simulink model "BMS_M0_pack_withoutcharging"  (R2026a)
settings: Solver=VariableStepAuto  AbsTol=1e-3  EnableMultiTasking=on
undefined symbols (not defined in the file or in its folder): bat, mcu
libraries: fl_lib x23, nesl_utility x19, batteryecm_lib x6, ee_lib x4, simulink x1
settings SimscapeCC: SimscapeNominalValues="[{\"value\":\"1\",\"unit\":\"A\"},{\"value\":\"1\",\"unit\":\"bar\"},{\"value\":\"1\",\"unit\":\"cm^2\"},{\"value\":\"1\",\"unit\":\"cm^3/s\"},{\"value\":\"1\",\"unit\":\"kJ/kg\"},{\"value\":\"1\",\"unit\":\"kW\"},{\"value\":\"1\",\"unit\":\"l\"},{\"value\":\"1\",\"unit\":\"N\"},{\"value\":\"1\",\"unit\":\"N*m\"},{\"value\":\"1\",\"unit\":\"V\"}]"

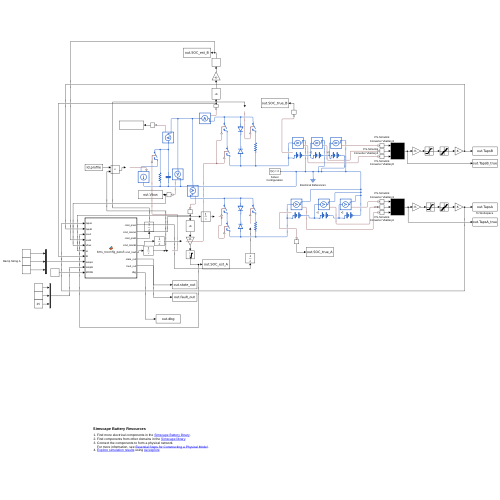
[thumbnail: Simulink's stored preview of the top-level diagram]
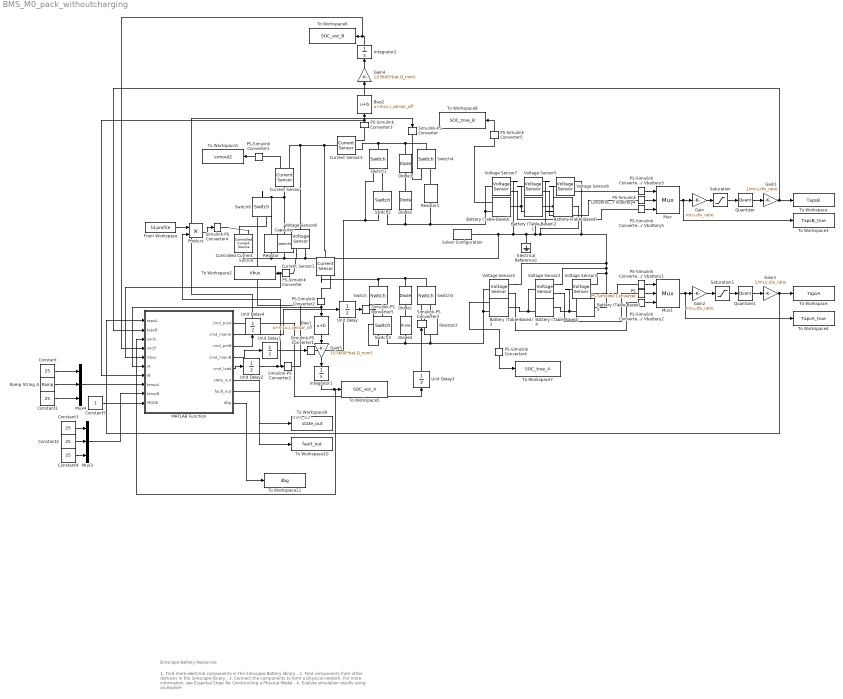
== system BMS_M0_pack_withoutcharging ==
  note: 1. Find more electrical components in the Simscape Battery library .
      | 2. Find components from other domains in the Simscape library .
      | 3. Connect the components to form a physical network.
      | For more information, see Essential Steps for Constructing a Physical Model .
      | 4. Explore simulation results using sscexplore
  note: Simscape Battery Resources
  note: state_out
  Battery (Table-Based){,1..5} (6 alike) : batteryecm_lib/Battery (Table-Based)  SOC_vec=bat.SOC_bp  T_dependence=simscape.enum.tablebattery.temperature_dependence.no  prm_dir=simscape.enum.tablebattery.prm_dir.noCurrentDirectionality  T_vec=[278, 293, 313] K  V0_mat=[3.49, 3.5, 3.51; 3.55, 3.57, 3.56; 3.62, 3.63, 3.64; 3.71, 3.71, 3.72; 3.91, 3.93, 3.94; 4.07, 4.08, 4.08; 4.19, 4.19, 4.19] V  V0_vec=bat.OCV_tbl V  V_range=[0, inf] V  R0_mat=[.0117, .0085, .009; .011, .0085, .009; .0114, .0087, .0092; .0107, .0082, .0088; .0107, .0083, .0091; .0113, .0085, .0089; .0116, .0085, .0089] Ohm  R0_vec=bat.R0 * ones(size(bat.SOC_bp)) Ohm  R0_dis_mat=[.0117, .0085, .009; .011, .0085, .009; .0114, .0087, .0092; .0107, .0082, .0088; .0107, .0083, .0091; .0113, .0085, .0089; .0116, .0085, .0089] Ohm  R0_dis_vec=[.0085, .0085, .0087, .0082, .0083, .0085, .0085] Ohm  R0_ch_mat=[.0117, .0085, .009; .011, .0085, .009; .0114, .0087, .0092; .0107, .0082, .0088; .0107, .0083, .0091; .0113, .0085, .0089; .0116, .0085, .0089] Ohm  R0_ch_vec=[.0085, .0085, .0087, .0082, .0083, .0085, .0085] Ohm  AH=bat.Q_nom A*hr  prm_leak=simscape.enum.tablebattery.prm_leak.disabled  Rleak_vec=[8000, 7000, 6000] Ohm  Rleak=7e3 Ohm  extrapolation_option=simscape.enum.extrapolation.nearest  SOC_port=simscape.enum.tablebattery.enable.yes  prm_dyn=simscape.enum.tablebattery.prm_dyn.off  R1_mat=[.0109, .0029, .0013; .0069, .0024, .0012; .0047, .0026, .0013; .0034, .0016, .001; .0033, .0023, .0014; .0033, .0018, .0011; .0028, .0017, .0011] Ohm  R1_vec=[.0029, .0024, .0026, .0016, .0023, .0018, .0017] Ohm  tau1_mat=[20, 36, 39; 31, 45, 39; 109, 105, 61; 36, 29, 26; 59, 77, 67; 40, 33, 29; 25, 39, 33] s  tau1_vec=[36, 45, 105, 29, 77, 33, 39] s  R2_mat=[.0109, .0029, .0013; .0069, .0024, .0012; .0047, .0026, .0013; .0034, .0016, .001; .0033, .0023, .0014; .0033, .0018, .0011; .0028, .0017, .0011] Ohm  R2_vec=[.0029, .0024, .0026, .0016, .0023, .0018, .0017] Ohm  tau2_mat=[20, 36, 39; 31, 45, 39; 109, 105, 61; 36, 29, 26; 59, 77, 67; 40, 33, 29; 25, 39, 33] s  tau2_vec=[36, 45, 105, 29, 77, 33, 39] s  R3_mat=[.0109, .0029, .0013; .0069, .0024, .0012; .0047, .0026, .0013; .0034, .0016, .001; .0033, .0023, .0014; .0033, .0018, .0011; .0028, .0017, .0011] Ohm  R3_vec=[.0029, .0024, .0026, .0016, .0023, .0018, .0017] Ohm  tau3_mat=[20, 36, 39; 31, 45, 39; 109, 105, 61; 36, 29, 26; 59, 77, 67; 40, 33, 29; 25, 39, 33] s  tau3_vec=[36, 45, 105, 29, 77, 33, 39] s  R4_mat=[.0109, .0029, .0013; .0069, .0024, .0012; .0047, .0026, .0013; .0034, .0016, .001; .0033, .0023, .0014; .0033, .0018, .0011; .0028, .0017, .0011] Ohm  R4_vec=[.0029, .0024, .0026, .0016, .0023, .0018, .0017] Ohm  tau4_mat=[20, 36, 39; 31, 45, 39; 109, 105, 61; 36, 29, 26; 59, 77, 67; 40, 33, 29; 25, 39, 33] s  tau4_vec=[36, 45, 105, 29, 77, 33, 39] s  R5_mat=[.0109, .0029, .0013; .0069, .0024, .0012; .0047, .0026, .0013; .0034, .0016, .001; .0033, .0023, .0014; .0033, .0018, .0011; .0028, .0017, .0011] Ohm  R5_vec=[.0029, .0024, .0026, .0016, .0023, .0018, .0017] Ohm  tau5_mat=[20, 36, 39; 31, 45, 39; 109, 105, 61; 36, 29, 26; 59, 77, 67; 40, 33, 29; 25, 39, 33] s  tau5_vec=[36, 45, 105, 29, 77, 33, 39] s  prm_fade=simscape.enum.tablebattery.prm_fade.disabled  N0=100  dV0=0  dR0=0  dAH=0  dRleak=0  dR1=0  dR2=0  dR3=0  dR4=0  dR5=0  N0vec=[0, 100, 200, 300]  Tfadevec=[298.15, 323.15] K  dV0vec=[0, 0, 0, 0]  dR0vec=[0, 0, 0, 0]  dAHvec=[0, 0, 0, 0]  dRleakvec=[0, 0, 0, 0]  dR1vec=[0, 0, 0, 0]  dR2vec=[0, 0, 0, 0]  dR3vec=[0, 0, 0, 0]  dR4vec=[0, 0, 0, 0]  dR5vec=[0, 0, 0, 0]  dV0mat=[0, 0; 0, 0; 0, 0; 0, 0]  dR0mat=[0, 0; 0, 0; 0, 0; 0, 0]  dAHmat=[0, 0; 0, 0; 0, 0; 0, 0]  dRleakmat=[0, 0; 0, 0; 0, 0; 0, 0]  dR1mat=[0, 0; 0, 0; 0, 0; 0, 0]  dR2mat=[0, 0; 0, 0; 0, 0; 0, 0]  dR3mat=[0, 0; 0, 0; 0, 0; 0, 0]  dR4mat=[0, 0; 0, 0; 0, 0; 0, 0]  dR5mat=[0, 0; 0, 0; 0, 0; 0, 0]  prm_age_modeling=simscape.enum.tablebattery.prm_age_modeling.equation  storage_dt_age_vec=[0] d  storage_T_age_vec=[273] K  prm_age_OCV=simscape.enum.tablebattery.prm_age_OCV.OCV  OCV_age=0.9  SOC_age=0.6  prm_age_resistance=simscape.enum.tablebattery.prm_age.disabled  OCV_scaling_age_resistance=2.2134e6  OCV_offset_age_resistance=1.632e6  temp_exp_age_resistance=0.515833569 V  t_exp_age_resistance=0.75  T_age_vec_resistance=[273.15, 298.15, 323.15] K  dt_age_vec_resistance=[0, 90, 180, 270] d  dR0_age_vec=[0, 0, 0]  t_meas_dR0_age=100 d  dR0_age_mat=[0, 0, 0; 0, 0, 0; 0, 0, 0; 0, 0, 0]  prm_age_capacity=simscape.enum.tablebattery.prm_age.disabled  OCV_scaling_age_capacity=1.5097e07  OCV_offset_age_capacity=8.3625e06  temp_exp_age_capacity=0.6011 V  t_exp_age_capacity=0.75  T_age_vec_capacity=[273.15, 298.15, 323.15] K  dt_age_vec_capacity=[0, 90, 180, 270] d  dAH_age_vec=[0, 0, 0]  t_meas_dAH_age=100 d  dAH_age_mat=[0, 0, 0; 0, 0, 0; 0, 0, 0; 0, 0, 0]  thermal_port=simscape.enum.thermaleffects.omit  temperature=298.15 K  thermal_mass=100 J/K  i_specify=off  i_priority=None  i=0 A  i_nominal_specify=off  i_nominal_value=1  i_nominal_unit=A  v_specify=off  v_priority=None  v=0 V  v_nominal_specify=off  v_nominal_value=1  v_nominal_unit=V  stateOfCharge_specify=on  stateOfCharge_priority=High  stateOfCharge=0.50  stateOfCharge_nominal_specify=off  stateOfCharge_nominal_value=1  stateOfCharge_nominal_unit=1  num_cycles_specify=off  num_cycles_priority=High  num_cycles=0  num_cycles_nominal_specify=off  num_cycles_nominal_value=1  num_cycles_nominal_unit=1  cell_temperature_specify=off  cell_temperature_priority=High  cell_temperature=298.15 K  cell_temperature_nominal_specify=off  cell_temperature_nominal_value=1  cell_temperature_nominal_unit=K
      settings: LibrarySourceBlock=|
      | batt_lib/Cells/Battery
      | (Table-Based)
  Bias1 : Bias  Bias=mcu.i_sensor_off  SaturateOnIntegerOverflow=off
  Bias2 : Bias  Bias=mcu.i_sensor_off  SaturateOnIntegerOverflow=off
  Capacitor : fl_lib/Electrical/Electrical Elements/Capacitor  c=1000 uF  r=1e-6 Ohm  g=0 1/Ohm  i_specify=off  i_priority=None  i=0 A  i_nominal_specify=off  i_nominal_value=1  i_nominal_unit=A  v_specify=off  v_priority=None  v=0 V  v_nominal_specify=off  v_nominal_value=1  v_nominal_unit=V  vc_specify=off  vc_priority=High  vc=0 V  vc_nominal_specify=off  vc_nominal_value=1  vc_nominal_unit=V
  Constant{,1..4} (5 alike) : Constant  Value=25
  Constant5 : Constant
  Controlled Current Source : fl_lib/Electrical/Electrical Sources/Controlled Current Source
  Current Sensor : fl_lib/Electrical/Electrical Sensors/Current Sensor
  Current Sensor1 : fl_lib/Electrical/Electrical Sensors/Current Sensor
  Current Sensor3 : fl_lib/Electrical/Electrical Sensors/Current Sensor
  Diode{1..4} (4 alike) : ee_lib/Semiconductors & Converters/Diode  ModelType=ee.enum.diode.modelType.pwl  TableType=ee.enum.diode.tableType.IfMat  IfMat=[.07, .12, .19, 1.75, 4.24, 7.32, 11.2; .16, .3, .72, 2.14, 5.02, 8.35, 13.12] A  VfMat=[.9, 1.15, 1.25, 1.5, 1.75, 2.17, 2.6, 2.85; .58, .68, .75, 1.1, 1.38, 1.77, 2.27, 2.7] V  TjVec=[25, 125] degC  VfVec=[.5, .7, .9, 1.3, 1.7, 2.1, 2.5] V  IfVec=[.1, .2, .5, 1, 2, 4, 7, 10] A  IrMat=[1e-06, 2e-06, 5e-06, 1e-05, 2.5e-05, 5e-05, .0001; 2e-06, 5e-06, 1e-05, 4e-05, 8e-05, .0002, .0005] A  VrMat=[10, 100, 200, 250, 300, 325, 350; 10, 70, 160, 220, 270, 300, 320] V  VrVec=[10, 20, 40, 50, 70, 80, 100] V  IrVec=[1e-06, 2e-06, 5e-06, 1e-05, 2e-05, 5e-05, .0001] A  Vf=0.8 V  Ron=0.01 Ohm  Goff=1e-8 S  prmExp=ee.enum.diode.expParam.useTwo  I12=[.0137, .545] A  V12=[.6, .7] V  RS=0 Ohm  Tmeas=298.15 K  IS=1e-12 A  ec=1  I1=0.0137 A  V1=0.6 V  N_series=1  N_parallel=1  ZenerEnable=false  Rz=0.3 Ohm  BV=30 V  C_param=ee.enum.diode.capParam.fixed  CJ=0 pF  CJ0=5 pF  Vvec=[.1, 10, 100] V  Cvec=[3.5, 1, .4] pF  VJ=1 V  Mgrad=0.5  FC=0.5  Q_param=ee.enum.diode.recoveryParam.off  iRM=-7.15 A  iF=4 A  didt=-750 A/us  trr_factor=3  trr=115 ns  Qrr=150 nA*s  Vr=-600 V  Ls=150 nH  Erec=0.03 J  TT=50 ns  tau=100 ns  T_param=ee.enum.diode.temperatureParam.off  Tdevice=298.15 K  I1_T2=0.245 A  V1_T2=0.5 V  IS_T2=1.25e-7 A  Tmeas2=125 degC  XTI_param=ee.enum.diode.xtiParam.pn  XTI=3  EG_param=ee.enum.diode.egapParam.material_si  EG=1.11 eV  dBVdT=0 V/K  enable_fault_input=simscape.enum.onoff.off  i_specify=off  i_priority=None  i=0 A  i_nominal_specify=off  i_nominal_value=1  i_nominal_unit=A  v_specify=off  v_priority=None  v=0 V  v_nominal_specify=off  v_nominal_value=1  v_nominal_unit=V  v_capacitor_specify=off  v_capacitor_priority=None  v_capacitor=0 V  v_capacitor_nominal_specify=off  v_capacitor_nominal_value=1  v_capacitor_nominal_unit=V  Qj_specify=off  Qj_priority=High  Qj=0 C  Qj_nominal_specify=off  Qj_nominal_value=1  Qj_nominal_unit=C  i_diode_specify=off  i_diode_priority=None  i_diode=0 A  i_diode_nominal_specify=off  i_diode_nominal_value=1  i_diode_nominal_unit=A  v_diode_specify=off  v_diode_priority=None  v_diode=0 V  v_diode_nominal_specify=off  v_diode_nominal_value=1  v_diode_nominal_unit=V  i_capacitor_specify=off  i_capacitor_priority=None  i_capacitor=0 A  i_capacitor_nominal_specify=off  i_capacitor_nominal_value=1  i_capacitor_nominal_unit=A  fidelity_level=ee.enum.diode.fidelity.includeChargeDyn  rec_loss_model=ee.enum.diode.reverseRecoveryModelTabulateUpTo3D.fixed  ErecVal=0 J  scaleWithIandV=true  ErecMat=zeros(2, 3) J  ErecMat3D=zeros(2, 3, 2) J  TjrecVec=[298.15, 398.15] K  IfrecVec=[.1, 1, 10] A  IrecVal=10 A  VrecVal=10 V  VrecVec=[0, 100] V  tFilter=1 / 1000 / 100 s  thermal_network_parameterization=ee.enum.thermalNetworkTopology.junctionCase  Rth=[0, 10] K/W  Rth_Cauer=[1, 3, 10] K/W  Rth_Foster=[.08, .14, .22, .16] K/W  thermal_mass_parameterization=ee.enum.thermalNetwork.timeconstant  thermal_mass=[0, 1] J/K  thermal_mass_Cauer=[.1, .3, 1] J/K  thermal_mass_Foster=[.001, .005, .05, .5] J/K  thermal_time_constant=[0, 10] s  thermal_time_constant_Cauer=[1, 3, 10] s  thermal_time_constant_Foster=[7e-05, .0007, .01, .08] s  thermal_mass_initial_temperatures=[25, 25] degC  thermal_mass_initial_temperatures_Cauer=[25, 25, 25] degC  junction_thermal_mass=0.01 J/K  Tvec_initial_Foster=[25, 25, 25, 25] degC  no_thermal_network=0  junction_temperature_specify=off  junction_temperature_priority=None  junction_temperature=25 degC  junction_temperature_nominal_specify=off  junction_temperature_nominal_value=1  junction_temperature_nominal_unit=degC
  Electrical Reference1 : fl_lib/Electrical/Electrical Elements/Electrical Reference
  From Workspace : FromWorkspace  VariableName=ld.profile
  Gain : Gain  Gain=mcu.div_ratio
  Gain1 : Gain  Gain=1/mcu.div_ratio
  Gain2 : Gain  Gain=mcu.div_ratio
  Gain3 : Gain  Gain=1/mcu.div_ratio
  Gain4 : Gain  Gain=1/(3600*bat.Q_nom)
  Gain5 : Gain  Gain=1/(3600*bat.Q_nom)
  Integrator1 : Integrator  InitialCondition=0.55  LimitOutput=on  UpperSaturationLimit=1  LowerSaturationLimit=0
  Integrator2 : Integrator  InitialCondition=0.55  LimitOutput=on  UpperSaturationLimit=1  LowerSaturationLimit=0
  MATLAB Function : MATLAB Function  TreatAsAtomicUnit=on  SystemSampleTime=0.1
  Mux{,1,3..4} (4 alike) : Mux  Inputs=3
  PS : nesl_utility/PS-Simulink Converter  PhysicalDomain=network_engine_domain  SubClassName=ps_output  LeftPortType=input  RightPortType=output  PseudoPeriodic=off  Frequencies=[]  VectorFormat=inherit  Unit=inherit  AffineConversion=off
  PS-Simulink Converter{,1..5} (6 alike) : nesl_utility/PS-Simulink Converter  PhysicalDomain=network_engine_domain  SubClassName=ps_output  LeftPortType=input  RightPortType=output  PseudoPeriodic=off  Frequencies=[]  VectorFormat=inherit  Unit=inherit  AffineConversion=off
  PS-Simulink Converter Vbattery{1..5} (5 alike) : nesl_utility/PS-Simulink Converter  PhysicalDomain=network_engine_domain  SubClassName=ps_output  LeftPortType=input  RightPortType=output  PseudoPeriodic=off  Frequencies=[]  VectorFormat=inherit  Unit=inherit  AffineConversion=off
  Product : Product
  Quantizer : Quantizer  QuantizationInterval=mcu.lsb_adc
  Quantizer1 : Quantizer  QuantizationInterval=mcu.lsb_adc
  Ramp String A : simulink/Sources/Ramp  slope=5/60  start=1e9  InitialOutput=25
  Resistor : fl_lib/Electrical/Electrical Elements/Resistor  R=1 MOhm  i_specify=off  i_priority=None  i=0 A  i_nominal_specify=off  i_nominal_value=1  i_nominal_unit=A  v_specify=off  v_priority=None  v=0 V  v_nominal_specify=off  v_nominal_value=1  v_nominal_unit=V
  Resistor1 : fl_lib/Electrical/Electrical Elements/Resistor  R=10 Ohm  i_specify=off  i_priority=None  i=0 A  i_nominal_specify=off  i_nominal_value=1  i_nominal_unit=A  v_specify=off  v_priority=None  v=0 V  v_nominal_specify=off  v_nominal_value=1  v_nominal_unit=V
  Resistor2 : fl_lib/Electrical/Electrical Elements/Resistor  R=10 Ohm  i_specify=off  i_priority=None  i=0 A  i_nominal_specify=off  i_nominal_value=1  i_nominal_unit=A  v_specify=off  v_priority=None  v=0 V  v_nominal_specify=off  v_nominal_value=1  v_nominal_unit=V
  Saturation : Saturate  UpperLimit=3.3  LowerLimit=0
  Saturation1 : Saturate  UpperLimit=3.3  LowerLimit=0
  Simulink-PS Converter{,1..5} (6 alike) : nesl_utility/Simulink-PS Converter  PhysicalDomain=network_engine_domain  SubClassName=ps_input  LeftPortType=input  RightPortType=output  PseudoPeriodic=off  Frequencies=[]  NoiseDistribution=none  NoiseParameters=[]  Unit=1  AffineConversion=off  FilteringAndDerivatives=provide  SimscapeFilterOrder=1  InputFilterTimeConstant=0.001  UdotUserProvided=0
  Solver Configuration : nesl_utility/Solver Configuration  PhysicalDomain=network_engine_domain  SubClassName=solver  LeftPortType=input  RightPortType=generic  Tones=[]  Harmonics=[]  SimulateNoise=off  Profile=off  UseLocalSampling=off  EnableSwitchedLinearOptims=on  FrequencyDomain=off  UseCCode=off  RelTol=0.001  AbsTol=1e-06  MinStep=1e-09  ToWorkspace=off  RevertToSquareIcSolve=off  NumHomotopyIterations=100  PhasorMode=off  PhasorModeNumHarmonics=1  ConsistencySolver=NEWTON_XTOL_AFTER_FTOL  CanonicalOrdering=UNORDERED  OptimizeIntermediates=UNOPTIMIZED  IndexReductionMethod=DerivativeReplacement  DoDC=off  ResidualTolerance=1e-09  ConsistencyTolSource=GLOBAL  ConsistencyAbsTol=0.001  ConsistencyRelTol=0.001  ConsistencyTolFactor=0.001  UseLocalSolver=off  LocalSolverChoice=NE_BACKWARD_EULER_ADVANCER  ResolveIndetEquations=on  FunctionEvalNumThread=1  LocalSolverSampleTime=0.001  DoFixedCost=off  MaxNonlinIter=3  MaxModeIter=2  ComputeImpulses=off  ImpulseIterations=2  LinearAlgebra=auto  LinearAlgebraNumThread=0  EquationFormulation=NE_TIME_EF  DelaysMemoryBudget=1024  AutomaticFiltering=on  FilteringTimeConstant=0.001  PartitionStorageMethod=AS_NEEDED  PartitionMemoryBudget=1024  PartitionMethod=ROBUST  MultibodyUseLocalSolver=off  MultibodyLocalSolverChoice=ODE1  MultibodyLocalSolverSampleTime=0.001
  Switch{,1..3,6} (5 alike) : fl_lib/Electrical/Electrical Elements/Switch  R_closed=fet.Rds_on Ohm  G_open=1e-8 1/Ohm  Threshold=0.5  i_specify=off  i_priority=None  i=0 A  i_nominal_specify=off  i_nominal_value=1  i_nominal_unit=A  v_specify=off  v_priority=None  v=0 V  v_nominal_specify=off  v_nominal_value=1  v_nominal_unit=V
  Switch4 : fl_lib/Electrical/Electrical Elements/Switch  R_closed=0.01 Ohm  G_open=1e-8 1/Ohm  Threshold=0.5  i_specify=off  i_priority=None  i=0 A  i_nominal_specify=off  i_nominal_value=1  i_nominal_unit=A  v_specify=off  v_priority=None  v=0 V  v_nominal_specify=off  v_nominal_value=1  v_nominal_unit=V
  Switch5 : fl_lib/Electrical/Electrical Elements/Switch  R_closed=0.01 Ohm  G_open=1e-8 1/Ohm  Threshold=0.5  i_specify=off  i_priority=None  i=0 A  i_nominal_specify=off  i_nominal_value=1  i_nominal_unit=A  v_specify=off  v_priority=None  v=0 V  v_nominal_specify=off  v_nominal_value=1  v_nominal_unit=V
  To Workspace : ToWorkspace  VariableName=TapsB  SaveFormat=Timeseries  SampleTime=-1
  "To Workspace " : ToWorkspace  VariableName=TapsA  SaveFormat=Timeseries  SampleTime=-1
  To Workspace1 : ToWorkspace  VariableName=simout2  SaveFormat=Timeseries  SampleTime=-1
  To Workspace10 : ToWorkspace  VariableName=fault_out  SaveFormat=Timeseries  SampleTime=-1
  To Workspace11 : ToWorkspace  VariableName=dbg  SaveFormat=Timeseries  SampleTime=-1
  To Workspace2 : ToWorkspace  VariableName=Vbus  SaveFormat=Timeseries  SampleTime=-1
  To Workspace3 : ToWorkspace  VariableName=TapsB_true  SaveFormat=Timeseries  SampleTime=-1
  To Workspace4 : ToWorkspace  VariableName=TapsA_true  SaveFormat=Timeseries  SampleTime=-1
  To Workspace5 : ToWorkspace  VariableName=SOC_est_A  SaveFormat=Timeseries  SampleTime=-1
  To Workspace6 : ToWorkspace  VariableName=SOC_est_B  SaveFormat=Timeseries  SampleTime=-1
  To Workspace7 : ToWorkspace  VariableName=SOC_true_A  SaveFormat=Timeseries  SampleTime=-1
  To Workspace8 : ToWorkspace  VariableName=SOC_true_B  SaveFormat=Timeseries  SampleTime=-1
  To Workspace9 : ToWorkspace  VariableName=state_out  SaveFormat=Timeseries  SampleTime=-1
  Unit Delay{,1..4} (5 alike) : UnitDelay  SampleTime=0.1
  Voltage Sensor{2..8} (7 alike) : fl_lib/Electrical/Electrical Sensors/Voltage Sensor
  wires:
  Saturation1/1 -> Quantizer1/1
  Unit Delay2/1 -> Product/2, Simulink-PS Converter2/1
  PS-Simulink Converter3/1 -> MATLAB Function/7(iB), Bias2/1
  Mux4/1 -> MATLAB Function/8(tempA)
  MATLAB Function/8(dbg) -> To Workspace11/1
  Constant1/1 -> Mux4/3
  Constant5/1 -> MATLAB Function/10(MODE)
  Unit Delay/1 -> Simulink-PS Converter5/1
  PS-Simulink Converter Vbattery3/1 -> Mux/1
  MATLAB Function/4(cmd_mainB) -> Unit Delay1/1
  PS-Simulink Converter Vbattery1/1 -> Mux1/1
  Ramp String A/1 -> Mux4/2
  Constant/1 -> Mux4/1
  Constant4/1 -> Mux3/3
  PS-Simulink Converter/1 -> To Workspace2/1, MATLAB Function/5(Vbus)
  PS-Simulink Converter2/1 -> MATLAB Function/6(iA), Bias1/1
  Product/1 -> Simulink-PS Converter4/1
  Quantizer1/1 -> Gain3/1
  MATLAB Function/3(cmd_preB) -> Unit Delay4/1
  Gain/1 -> Saturation/1
  PS-Simulink Converter5/1 -> To Workspace8/1
  Quantizer/1 -> Gain1/1
  Constant3/1 -> Mux3/1
  PS-Simulink Converter Vbattery5/1 -> Mux/3
  Integrator2/1 -> MATLAB Function/4(socB), To Workspace6/1
  Saturation/1 -> Quantizer/1
  Bias2/1 -> Gain4/1
  Integrator1/1 -> To Workspace5/1, MATLAB Function/3(socA)
  Unit Delay3/1 -> Simulink-PS Converter3/1
  Mux3/1 -> MATLAB Function/9(tempB)
  PS-Simulink Converter1/1 -> To Workspace1/1
  MATLAB Function/5(cmd_load) -> Unit Delay2/1
  MATLAB Function/6(state_out) -> To Workspace9/1
  MATLAB Function/2(cmd_mainA) -> Unit Delay/1
  Gain5/1 -> Integrator1/1
  PS-Simulink Converter Vbattery4/1 -> Mux/2
  From Workspace/1 -> Product/1
  Gain1/1 -> To Workspace/1, MATLAB Function/2(tapsB)
  Gain4/1 -> Integrator2/1
  Gain3/1 -> "To Workspace "/1, MATLAB Function/1(tapsA)
  Constant2/1 -> Mux3/2
  PS-Simulink Converter Vbattery2/1 -> Mux1/3
  Unit Delay1/1 -> Simulink-PS Converter1/1
  PS-Simulink Converter4/1 -> To Workspace7/1
  PS/1 -> Mux1/2
  Mux/1 -> To Workspace3/1, Gain/1
  Gain2/1 -> Saturation1/1
  MATLAB Function/7(fault_out) -> To Workspace10/1
  MATLAB Function/1(cmd_preA) -> Unit Delay3/1
  Mux1/1 -> To Workspace4/1, Gain2/1
  Unit Delay4/1 -> Simulink-PS Converter/1
  Bias1/1 -> Gain5/1
  connections:
  Voltage Sensor6/RConn2 -- Battery (Table-Based)5/RConn1 -- Voltage Sensor3/RConn2 -- Voltage Sensor2/RConn2 -- Voltage Sensor4/RConn2 -- Solver Configuration/RConn1 -- Controlled Current Source/LConn1 -- Resistor/RConn1 -- Capacitor/RConn1 -- Voltage Sensor8/RConn2 -- Voltage Sensor7/RConn2 -- Electrical Reference1/LConn1 -- Voltage Sensor5/RConn2 -- Battery (Table-Based)2/RConn1
  Diode1/LConn1 -- Switch/LConn1 -- Current Sensor1/RConn2 -- Switch5/LConn1
  Current Sensor3/RConn2 -- Switch1/LConn1 -- Switch4/LConn1 -- Diode3/LConn1
  Switch/RConn1 -- Simulink-PS Converter5/RConn1 -- Switch3/RConn1
  Battery (Table-Based)2/LConn1 -- Battery (Table-Based)1/RConn1 -- Voltage Sensor6/LConn1
  Battery (Table-Based)5/LConn1 -- Battery (Table-Based)4/RConn1 -- Voltage Sensor3/LConn1
  Diode2/LConn1 -- Switch2/RConn2 -- Resistor1/RConn1 -- Voltage Sensor7/LConn1 -- Battery (Table-Based)/LConn1
  Switch2/RConn1 -- Simulink-PS Converter1/RConn1 -- Switch1/RConn1
  Current Sensor/RConn2 -- Current Sensor3/LConn1 -- Current Sensor1/LConn1 -- Voltage Sensor8/LConn1
  Voltage Sensor4/LConn1 -- Resistor2/RConn1 -- Diode4/LConn1 -- Switch3/RConn2 -- Battery (Table-Based)3/LConn1
  Battery (Table-Based)4/LConn1 -- Battery (Table-Based)3/RConn1 -- Voltage Sensor2/LConn1
  Switch6/LConn1 -- Capacitor/LConn1 -- Current Sensor/LConn1 -- Resistor/LConn1
  Voltage Sensor5/LConn1 -- Battery (Table-Based)/RConn1 -- Battery (Table-Based)1/LConn1
  Voltage Sensor6/RConn1 -- PS-Simulink Converter Vbattery3/LConn1
  Simulink-PS Converter3/RConn1 -- Switch5/RConn1
  Switch1/RConn2 -- Switch2/LConn1
  Current Sensor3/RConn1 -- PS-Simulink Converter3/LConn1
  Voltage Sensor4/RConn1 -- PS-Simulink Converter Vbattery2/LConn1
  Current Sensor/RConn1 -- PS-Simulink Converter1/LConn1
  Resistor1/LConn1 -- Switch4/RConn2
  Voltage Sensor8/RConn1 -- PS-Simulink Converter/LConn1
  Switch6/RConn2 -- Controlled Current Source/RConn2
  Switch/RConn2 -- Switch3/LConn1
  Simulink-PS Converter2/RConn1 -- Switch6/RConn1
  PS-Simulink Converter4/LConn1 -- Battery (Table-Based)3/LConn2
  Simulink-PS Converter4/RConn1 -- Controlled Current Source/RConn1
  Voltage Sensor5/RConn1 -- PS-Simulink Converter Vbattery4/LConn1
  Diode4/RConn1 -- Diode1/RConn1
  Resistor2/LConn1 -- Switch5/RConn2
  Voltage Sensor3/RConn1 -- PS-Simulink Converter Vbattery1/LConn1
  Voltage Sensor2/RConn1 -- PS/LConn1
  Current Sensor1/RConn1 -- PS-Simulink Converter2/LConn1
  Voltage Sensor7/RConn1 -- PS-Simulink Converter Vbattery5/LConn1
  Battery (Table-Based)/LConn2 -- PS-Simulink Converter5/LConn1
  Diode2/RConn1 -- Diode3/RConn1
  Switch4/RConn1 -- Simulink-PS Converter/RConn1

== matlab function BMS_M0_pack_withoutcharging/MATLAB Function ==
  data: cmd_preA output; tapsA input; cmd_mainA output; cmd_preB output; tapsB input; socA input; socB input; cmd_mainB output; cmd_load output; state_out output; fault_out output; Vbus input; iA input; iB input; dbg output; tempA input; tempB input; MODE input
function [cmd_preA, cmd_mainA, cmd_preB, cmd_mainB, cmd_load, ...
          state_out, fault_out, dbg] = ...
         bms_reconfig_pass5(tapsA, tapsB, socA, socB, Vbus, iA, iB, ...
                            tempA, tempB, MODE)
%BMS_RECONFIG_PASS5  SOC/SOA-driven string-level reconfiguration controller.
%
%  ====================================================================
%  PROPRIETARY -- this file contains the novel contribution of this
%  project: dynamic string connect/disconnect/precharge for fault
%  isolation and SOC-driven wear levelling in a reconfigurable 3S2P pack.
%  Do not paste this logic into generic BMS code templates.
%  ====================================================================
%
%  MILESTONE 0 -- PASS 5 (final for M0).
%
%  REVISION HISTORY
%    Rev 1  SOA + topology logic.
%    Rev 2  Weld detection gated on precharge (Rev 1 tripped F_WELD_A on
%           startup because precharge current flows while the main pair is
%           deliberately open). SOC rejoin hysteresis actually applied --
%           Rev 1 rejoined at gap <= SPLIT_TH instead of < REJOIN_TH, so
%           the hysteresis band did nothing.
%    Rev 3  Warm-parallel guard reformulated. The 0.1 V rule is retained
%           for cold start, but under load the terminal difference between
%           strings is dominated by IR drop rather than stored-energy
%           mismatch, so it can never be satisfied. Bounded inrush is the
%           physically meaningful criterion. MEASURED Scenario 3: join at
%           dV = 0.149 V, inrush 1.5 A -> I_JOIN_MAX = 6 A gives 4x margin
%           while still blocking the 6.9 A cold-parallel case.
%    Rev 4  Overtemperature added.
%    Rev 5  MODE input added for the Day 5 fixed-vs-reconfigurable
%           comparison. The override MUST sit after the transition switch
%           statement -- an earlier attempt placed it before, where it was
%           silently overwritten by `case S_BOTH` within the same call and
%           the two configurations produced identical results.
%
%  DESIGN RULES (from project brief, enforced in this order):
%    1. SOA checks run BEFORE any efficiency or balancing logic.
%    2. Break-before-make on every topology change.
%    3. Never parallel two strings unless the resulting inrush is bounded
%       (see Rev 3 note -- the original 0.1 V form is kept for cold start).
%    4. Minimum cooldown between topology changes (anti-oscillation).
%    5. Power-up / reset default is ALL SWITCHES OPEN.
%    6. Every switching action is validated by reading back current.
%
%  INPUTS
%    tapsA, tapsB  3x1  quantised tap voltages, referenced to pack negative
%    socA, socB    1x1  COULOMB-COUNTED estimates. Never true SOC.
%    Vbus          1x1  bus voltage (measured)
%    iA, iB        1x1  per-string current (measured, + = discharge)
%    tempA, tempB  3x1  per-cell temperature (deg C).
%                       INJECTED forcing function, not a thermal model --
%                       see M0 Day 1 scope decision. M0 makes NO claim
%                       about temperature reduction; that is bench-measured
%                       in M4.
%    MODE          1x1  0 = fixed-pack baseline, 1 = reconfigurable.
%                       See the MODE block in LAYER 3 for what MODE 0
%                       does and why the comparison is fair.
%
%  OUTPUTS
%    cmd_preA/B    0/1  precharge bypass switch per string
%    cmd_mainA/B   0/1  main back-to-back pair per string
%    cmd_load      0/1  load disconnect switch
%    state_out          state code
%    fault_out          latched fault bitfield
%    dbg          10x1  diagnostics

%% ---- CONSTANTS ------------------------------------------------------
% KEEP IN SYNC WITH BMS_params.m -- a MATLAB Function block cannot read
% the base workspace.
DT              = 0.100;  % s   control loop period
V_UV_TRIP       = 2.50;   % V   [VERIFIED] SPEC pack design guideline, NCA
V_OV_TRIP       = 4.20;   % V   [VERIFIED] SPEC 3.3
I_OC_TRIP       = 12.0;   % A   [ASSUMPTION] per string, below the 15 A
                          %     cell rating with margin
T_OT_TRIP       = 60.0;   % C   [DESIGN] SPEC recommends re-discharge
                          %     release below 60 C. INTRO p.6 shows a 10 A
                          %     discharge reaching 60.9 C -- i.e. exactly
                          %     the single-string fault-mode operating
                          %     point, so this threshold is meaningful
                          %     rather than arbitrary.
T_OT_WARN       = 50.0;   % C   [ASSUMPTION] early-warning margin
DV_PARALLEL_MAX = 0.10;   % V   [ASSUMPTION] cold-start parallel limit
I_JOIN_MAX      = 6.0;    % A   [MEASURED-derived] Scenario 3 joined at
                          %     1.5 A; 6 A is 4x that and still blocks the
                          %     6.9 A unbalanced-warm-join case
R_STRING        = 0.100;  % ohm [CALCULATED] 3*20 mOhm cells + 2*20 mOhm
                          %     back-to-back MOSFET pair
T_COOLDOWN      = 0.50;   % s   [ASSUMPTION] min between topology changes
T_PRECHARGE_MAX = 0.50;   % s   [CALCULATED] 5*tau = 50 ms at R_pre = 10
                          %     ohm, C_bus = 1000 uF; 10x margin
VBUS_PRE_FRAC   = 0.95;   % fraction of string voltage = precharge done
SOC_SPLIT_TH    = 0.15;   % [DESIGN] gap at which we stop paralleling
SOC_REJOIN_TH   = 0.05;   % [DESIGN] hysteresis band for rejoining
DEBOUNCE_N      = 3;      % consecutive samples before a fault latches
VALIDATE_N      = 5;      % samples allowed for a switch to prove it moved
I_CONDUCT_MIN   = 0.20;   % A   above this counts as "current flowing"
STARTUP_N       = 10;     % ignore SOA for first 1 s while Simscape settles

%% ---- STATE CODES ----------------------------------------------------
S_INIT     = 0;   S_PRE_A    = 1;   S_PRE_B    = 2;
S_SINGLE_A = 3;   S_SINGLE_B = 4;   S_BOTH     = 5;
S_SHUTDOWN = 6;

%% ---- FAULT BITS -----------------------------------------------------
F_NONE   = 0;
F_UV_A   = 1;     F_UV_B   = 2;
F_OV_A   = 4;     F_OV_B   = 8;
F_OC_A   = 16;    F_OC_B   = 32;
F_PRE_A  = 64;    F_PRE_B  = 128;
F_WELD_A = 256;   F_WELD_B = 512;
F_OPEN_A = 1024;  F_OPEN_B = 2048;
F_OT_A   = 4096;  F_OT_B   = 8192;    % overtemperature

%% ---- PERSISTENT STATE ----------------------------------------------
persistent state fault
persistent uvA_c uvB_c ovA_c ovB_c ocA_c ocB_c otA_c otB_c
persistent t_state t_cool startup_c
persistent last_mainA last_mainB last_preA last_preB validate_cA validate_cB

if isempty(state)
    % POWER-UP DEFAULT: everything open. Mirrors the 100k base pull-downs
    % on the 2N2222A drivers -- on reset or brownout the hardware holds
    % the MOSFETs off, and the controller agrees.
    state = S_INIT;  fault = F_NONE;
    uvA_c = 0; uvB_c = 0; ovA_c = 0; ovB_c = 0;
    ocA_c = 0; ocB_c = 0; otA_c = 0; otB_c = 0;
    t_state = 0; t_cool = 0; startup_c = 0;
    last_mainA = 0; last_mainB = 0;
    last_preA  = 0; last_preB  = 0;
    validate_cA = 0; validate_cB = 0;
end

startup_c = startup_c + 1;
t_state   = t_state + DT;
if t_cool > 0, t_cool = t_cool - DT; end

%% ---- RECONSTRUCT PER-CELL VOLTAGES ---------------------------------
% The firmware performs this same subtraction: the dividers measure taps
% relative to pack negative, not individual cells. Measured reconstruction
% error 0.39 mV typical, ~7 mV worst case (2 LSB at 3.46 mV/LSB).
vA = [ tapsA(1); tapsA(2)-tapsA(1); tapsA(3)-tapsA(2) ];
vB = [ tapsB(1); tapsB(2)-tapsB(1); tapsB(3)-tapsB(2) ];

vStringA = tapsA(3);
vStringB = tapsB(3);

tMaxA = max(tempA);
tMaxB = max(tempB);

%% ---- STARTUP GRACE --------------------------------------------------
if startup_c < STARTUP_N
    cmd_preA = 0; cmd_mainA = 0;
    cmd_preB = 0; cmd_mainB = 0; cmd_load = 0;
    state_out = S_INIT; fault_out = F_NONE;
    dbg = [vA(1); vA(2); vA(3); vB(1); vB(2); vB(3); 0; 0; tMaxA; tMaxB];
    return
end

%% =====================================================================
%  LAYER 1 -- SOA CHECKS. These run first, always, and override
%  everything below.
%  =====================================================================
if any(vA < V_UV_TRIP),  uvA_c = uvA_c + 1; else, uvA_c = 0; end
if any(vB < V_UV_TRIP),  uvB_c = uvB_c + 1; else, uvB_c = 0; end
if any(vA > V_OV_TRIP),  ovA_c = ovA_c + 1; else, ovA_c = 0; end
if any(vB > V_OV_TRIP),  ovB_c = ovB_c + 1; else, ovB_c = 0; end
if abs(iA) > I_OC_TRIP,  ocA_c = ocA_c + 1; else, ocA_c = 0; end
if abs(iB) > I_OC_TRIP,  ocB_c = ocB_c + 1; else, ocB_c = 0; end
if tMaxA   > T_OT_TRIP,  otA_c = otA_c + 1; else, otA_c = 0; end
if tMaxB   > T_OT_TRIP,  otB_c = otB_c + 1; else, otB_c = 0; end

% Faults LATCH. An unloaded cell recovers voltage and would look healthy
% again; a cell removed from a heat source cools. Re-closing on either
% would oscillate the pack.
if uvA_c >= DEBOUNCE_N, fault = bitor(fault, F_UV_A); end
if uvB_c >= DEBOUNCE_N, fault = bitor(fault, F_UV_B); end
if ovA_c >= DEBOUNCE_N, fault = bitor(fault, F_OV_A); end
if ovB_c >= DEBOUNCE_N, fault = bitor(fault, F_OV_B); end
if ocA_c >= DEBOUNCE_N, fault = bitor(fault, F_OC_A); end
if ocB_c >= DEBOUNCE_N, fault = bitor(fault, F_OC_B); end
if otA_c >= DEBOUNCE_N, fault = bitor(fault, F_OT_A); end
if otB_c >= DEBOUNCE_N, fault = bitor(fault, F_OT_B); end

%% ---- STATE VALIDATION ----------------------------------------------
% A MOSFET welded closed is invisible to voltage sensing -- only current
% reveals it. Gate on the PREVIOUS cycle's precharge command: while a
% precharge switch is closed the main pair is deliberately open yet
% current legitimately flows through R_pre, which is otherwise
% indistinguishable from a weld.
in_precharge = (last_preA == 1) || (last_preB == 1);

if ~in_precharge && last_mainA == 0 && abs(iA) > I_CONDUCT_MIN
    fault = bitor(fault, F_WELD_A);
end
if ~in_precharge && last_mainB == 0 && abs(iB) > I_CONDUCT_MIN
    fault = bitor(fault, F_WELD_B);
end
% Commanded closed but no current.
% Two fixes from M0 review:
%   (a) Split counters -- shared validate_c cross-contaminated A/B.
%   (b) Gate on evidence that current SHOULD be flowing:
%       S_BOTH:     other string is carrying current (proves load is active)
%       S_SINGLE_X: Vbus not tracking string voltage (proves switch isn't conducting)
%       Without this gate, a healthy no-load idle trips the detector.

i_total = abs(iA) + abs(iB);
vbus_tracks_A = (abs(Vbus - vStringA) < 1.0);
vbus_tracks_B = (abs(Vbus - vStringB) < 1.0);

% --- String A open-wire check ---
openA_cond = false;
if state == S_BOTH && last_mainA == 1 && ...
        abs(iA) < I_CONDUCT_MIN && i_total > I_CONDUCT_MIN && t_state > 1.0
    openA_cond = true;   % load is active but A carries nothing
elseif state == S_SINGLE_A && last_mainA == 1 && ...
        abs(iA) < I_CONDUCT_MIN && ~vbus_tracks_A && t_state > 1.0
    openA_cond = true;   % bus isn't tracking string A despite switch closed
end

if openA_cond
    validate_cA = validate_cA + 1;
    if validate_cA >= VALIDATE_N, fault = bitor(fault, F_OPEN_A); end
else
    validate_cA = 0;
end

% --- String B open-wire check ---
openB_cond = false;
if state == S_BOTH && last_mainB == 1 && ...
        abs(iB) < I_CONDUCT_MIN && i_total > I_CONDUCT_MIN && t_state > 1.0
    openB_cond = true;
elseif state == S_SINGLE_B && last_mainB == 1 && ...
        abs(iB) < I_CONDUCT_MIN && ~vbus_tracks_B && t_state > 1.0
    openB_cond = true;
end

if openB_cond
    validate_cB = validate_cB + 1;
    if validate_cB >= VALIDATE_N, fault = bitor(fault, F_OPEN_B); end
else
    validate_cB = 0;
end

faultA = bitand(fault, F_UV_A + F_OV_A + F_OC_A + F_OT_A + ...
                       F_PRE_A + F_WELD_A + F_OPEN_A) ~= 0;
faultB = bitand(fault, F_UV_B + F_OV_B + F_OC_B + F_OT_B + ...
                       F_PRE_B + F_WELD_B + F_OPEN_B) ~= 0;

%% =====================================================================
%  LAYER 2 -- BALANCING PREFERENCE (secondary; never overrides Layer 1)
%
%  A 2S string cannot be paralleled with a 3S string, so per-cell bypass
%  is unavailable. String-level selection is the only lever: run the
%  fuller string alone and let the emptier one rest.
%
%  MEASURED BEHAVIOUR (Scenario 3): from a 15% gap, single-string
%  operation closed the gap to 5% in 224 s, at which point the strings
%  rejoined. After rejoining the gap continued to zero WITHOUT controller
%  action -- paralleled strings self-balance through the bus. The value of
%  the split is therefore SAFE CONNECTION of mismatched strings, not extra
%  extracted energy. Do not claim the latter.
%  =====================================================================
soc_gap = socA - socB;
prefer_A_only = (soc_gap >  SOC_SPLIT_TH);
prefer_B_only = (soc_gap < -SOC_SPLIT_TH);
rejoin_ok     = (abs(soc_gap) < SOC_REJOIN_TH);

%% =====================================================================
%  LAYER 3 -- TRANSITION GUARDS
%  =====================================================================
% Cold start (load off, bus near 0 V): terminal dV is the right check.
% Warm parallel (load on): terminal dV is dominated by IR drop from the
% loaded string, not by stored-energy mismatch, so it can never fall below
% 0.1 V. Bound the resulting inrush instead -- that is the quantity the
% original rule was a proxy for.
dV_terminal = abs(vStringA - vStringB);
inrush_est  = dV_terminal / R_STRING;
dV_ok       = (dV_terminal < DV_PARALLEL_MAX) || (inrush_est < I_JOIN_MAX);

cool_ok   = (t_cool <= 0);
new_state = state;

switch state

    case S_INIT
        if     faultA && faultB, new_state = S_SHUTDOWN;
        elseif ~faultA,          new_state = S_PRE_A;
        elseif ~faultB,          new_state = S_PRE_B;
        else,                    new_state = S_SHUTDOWN;
        end

    case S_PRE_A
        % Bus charges through R_pre with the load disconnected. Only once
        % it has risen does the main pair close -- this is what keeps the
        % handover near 1 A instead of the measured 219 A cold-connect.
        if faultA
            new_state = S_SHUTDOWN;
        elseif Vbus >= VBUS_PRE_FRAC * vStringA
            new_state = S_SINGLE_A;
        elseif t_state > T_PRECHARGE_MAX
            fault = bitor(fault, F_PRE_A);
            new_state = S_SHUTDOWN;
        end

    case S_PRE_B
        if faultB
            new_state = S_SINGLE_A;
        elseif Vbus >= VBUS_PRE_FRAC * vStringB
            new_state = S_BOTH;
        elseif t_state > T_PRECHARGE_MAX
            fault = bitor(fault, F_PRE_B);
            new_state = S_SINGLE_A;
        end

    case S_SINGLE_A
        if     faultA && faultB,      new_state = S_SHUTDOWN;
        elseif faultA,                new_state = S_PRE_B;
        elseif ~faultB && cool_ok && dV_ok && rejoin_ok
                                      new_state = S_PRE_B;
        end

    case S_SINGLE_B
        if     faultA && faultB,      new_state = S_SHUTDOWN;
        elseif faultB,                new_state = S_PRE_A;
        elseif ~faultA && cool_ok && dV_ok && rejoin_ok
                                      new_state = S_PRE_A;
        end

    case S_BOTH
        if     faultA && faultB,         new_state = S_SHUTDOWN;
        elseif faultA,                   new_state = S_SINGLE_B;
        elseif faultB,                   new_state = S_SINGLE_A;
        elseif cool_ok && prefer_A_only, new_state = S_SINGLE_A;
        elseif cool_ok && prefer_B_only, new_state = S_SINGLE_B;
        end

    case S_SHUTDOWN
        % TERMINAL. Auto-recovery from an unknown fault is not defensible.

    otherwise
        new_state = S_SHUTDOWN;
end

%% ---- MODE 0: FIXED-PACK BASELINE ------------------------------------
% A conventional hard-paralleled pack has no string switches, so it cannot
% isolate a faulted string. Once both strings are connected the topology is
% frozen: faults still latch and are logged, but produce no reconfiguration.
% The only exit is total shutdown once the pack can no longer supply.
%
% Everything else -- cell models, switch resistance, body diodes, sensing,
% quantisation, precharge at startup -- is IDENTICAL to MODE 1. The only
% difference is the control policy, which is exactly what we are comparing.
%
% PLACEMENT MATTERS: this must run AFTER the switch statement above, so it
% overrides the new_state that `case S_BOTH` just computed. Placing it
% before the switch has no effect -- the transition logic simply recomputes
% new_state and the override is lost.
if MODE < 0.5 && state == S_BOTH
    if faultA && faultB
        new_state = S_SHUTDOWN;   % pack exhausted; nothing left to do
    else
        new_state = S_BOTH;       % freeze -- no isolation available
    end
end

if new_state ~= state
    state   = new_state;
    t_state = 0;
    t_cool  = T_COOLDOWN;
end

%% ---- OUTPUTS -------------------------------------------------------
% BREAK-BEFORE-MAKE is structural: no state asserts a precharge switch and
% its own main pair simultaneously.
switch state
    case S_INIT
        cmd_preA=0; cmd_mainA=0; cmd_preB=0; cmd_mainB=0; cmd_load=0;
    case S_PRE_A
        cmd_preA=1; cmd_mainA=0; cmd_preB=0; cmd_mainB=0; cmd_load=0;
    case S_SINGLE_A
        cmd_preA=0; cmd_mainA=1; cmd_preB=0; cmd_mainB=0; cmd_load=1;
    case S_PRE_B
        cmd_preA=0; cmd_mainA=1; cmd_preB=1; cmd_mainB=0; cmd_load=1;
    case S_SINGLE_B
        cmd_preA=0; cmd_mainA=0; cmd_preB=0; cmd_mainB=1; cmd_load=1;
    case S_BOTH
        cmd_preA=0; cmd_mainA=1; cmd_preB=0; cmd_mainB=1; cmd_load=1;
    case S_SHUTDOWN
        cmd_preA=0; cmd_mainA=0; cmd_preB=0; cmd_mainB=0; cmd_load=0;
    otherwise
        cmd_preA=0; cmd_mainA=0; cmd_preB=0; cmd_mainB=0; cmd_load=0;
end

last_mainA = cmd_mainA;  last_mainB = cmd_mainB;
last_preA  = cmd_preA;   last_preB  = cmd_preB;

state_out = state;
fault_out = fault;
dbg = [vA(1); vA(2); vA(3); vB(1); vB(2); vB(3); ...
       soc_gap; Vbus; tMaxA; tMaxB];

end

%% =====================================================================
%  FMEA -- PASS 5
%  =====================================================================
%
%  FAILURE                   DETECTION                   SAFE RESPONSE
%  --------------------------------------------------------------------
%  Cell undervoltage         cell < 2.50 V, 3 samples    Isolate string
%  Cell overvoltage          cell > 4.20 V, 3 samples    Isolate string
%  String overcurrent        |i| > 12 A, 3 samples       Isolate string
%  Cell overtemperature      T > 60 C, 3 samples         Isolate string
%
%  Internal cell short       Manifests as UV on that     Isolate string.
%  (the case a hard-          cell, and/or OT            Series topology
%   paralleled pack                                      means no loop
%   cannot address)                                      exists once the
%                                                        string switch is
%                                                        open. Measured
%                                                        leakage with the
%                                                        pair open:
%                                                        0.0004 mA.
%
%  MOSFET welded closed      commanded open but          Latch F_WELD;
%                            |i| > 0.2 A and not         cannot isolate,
%                            during precharge            so SHUTDOWN via
%                                                        load disconnect
%
%  MOSFET failed open        commanded closed but        Latch F_OPEN,
%                            |i| < 0.2 A, 5 samples      treat string as
%                                                        faulted
%
%  Single switch instead     N/A -- design-time.         MEASURED: a single
%  of a back-to-back pair    Body diode conducts.        switch leaked
%                                                        168,571 mA vs
%                                                        0.0004 mA for the
%                                                        pair. This is why
%                                                        the pair is
%                                                        mandatory.
%
%  Precharge resistor open   Vbus below 95% after        Latch F_PRE; do
%                            500 ms                      not close the main
%                                                        pair. Prevents the
%                                                        measured 218.8 A
%                                                        cold-connect.
%
%  Precharge switch welded   R_pre dissipates            NOT DETECTED.
%                            continuously                 [GAP -- needs a
%                                                        thermistor on
%                                                        R_pre or a
%                                                        separate i_pre
%                                                        measurement]
%
%  Both strings faulted      faultA && faultB            SHUTDOWN, load
%                                                        disconnected
%
%  Topology oscillation      T_COOLDOWN 500 ms +          Bounded to <= 2
%                            15%/5% SOC hysteresis        changes/second.
%                                                        MEASURED Scenario
%                                                        3: 6 transitions
%                                                        in 60 min.
%
%  Unsafe parallel join      inrush_est >= 6 A blocks    Transition blocked
%                            the transition               until the gap
%                                                        closes. MEASURED
%                                                        join: 1.5 A.
%
%  MCU reset mid-mission     persistents cleared          Re-enters S_INIT,
%                                                        all switches open;
%                                                        100k pull-downs
%                                                        hold the hardware
%                                                        off through reset
%
%  Coulomb counter drift     NOT DETECTED                 [KNOWN LIMITATION]
%                                                        MEASURED 5.06%
%                                                        after 10 min. SOC
%                                                        logic is secondary
%                                                        to SOA, so drift
%                                                        degrades balancing
%                                                        but never safety.
%
%  Capacity-fade lockout     NOT DETECTED                 [KNOWN GAP -- see
%  If one string accumulates                              below. Identified
%  more cycles its capacity                               during M0 review;
%  fades, so it reaches a                                 not yet mitigated]
%  given SOC faster. If the
%  capacities diverge far
%  enough the strings may
%  never satisfy rejoin_ok
%  simultaneously and the
%  pack locks permanently
%  into single-string
%  operation at half power.
%
%  KNOWN GAPS (M1 and beyond):
%    - Capacity-fade lockout, above. Mitigations to evaluate: track
%      cumulative Ah per string and favour the less-used string; or
%      compare capacity-normalised SOC rather than raw SOC in rejoin_ok.
%    - Precharge switch stuck-closed undetectable.
%    - Deliberate wear-levelling alternation not implemented. The SOC
%      split provides incidental alternation but is not driven by
%      cycle count.
%    - No thermal model. Temperature is an injected forcing function, so
%      M0 makes NO claim about temperature reduction. That is measured on
%      the bench in M4.
%    - Soft cell degradation is handled WORSE than a hard-paralleled pack:
%      isolating one weak cell costs the two healthy cells in its string.
%      State this trade-off explicitly rather than claiming general
%      superiority.
